simulink model "gm_cosim_fir_mq"  (R2015b)
settings: Solver=FixedStepDiscrete  SolverMode=SingleTasking  StartTime=0.0  StopTime=10.0  RelTol=1e-3
libraries: simulink x2, modelsimlib x1
settings Model: Creator=at-mt  LastModifiedBy=amatsumo
settings DataIOCC: SaveFormat=Array  SignalLoggingSaveFormat=ModelDataLogs  SaveOutput=off  SignalLogging=off  SaveTime=off
settings OptimizationCC: DefaultParameterBehavior=Inlined  ExpressionDepthLimit=2147483647
settings DebuggingCC: AlgebraicLoopMsg=error  UnderspecifiedInitializationDetection=Classic  MergeDetectMultiDrivingBlocksExec=none  SolverPrmCheckMsg=warning  InheritedTsInSrcMsg=none  SingleTaskRateTransMsg=error  ParameterPrecisionLossMsg=none  ParameterTunabilityLossMsg=none  FcnCallInpInsideContextMsg=UseLocalSettings  StateNameClashWarn=warning  StrictBusMsg=Warning
settings HardwareCC: ProdBitPerPointer=32  ProdLargestAtomicFloat=None  ProdIntDivRoundTo=Undefined  ProdEndianess=Unspecified  ProdWordSize=32  ProdHWDeviceType=ASIC/FPGA->ASIC/FPGA  ProdEqTarget=off
settings ModelReferenceCC: UpdateModelReferenceTargets=IfOutOfDate
settings SFSimCC: SFSimEcho=off
settings GRTTargetCC: GeneratePreprocessorConditionals=Disable all  CombineOutputUpdateFcns=off  GRTInterface=on
settings ConfigComp: CovModelRefEnable=Off  CovSFcnEnable=off

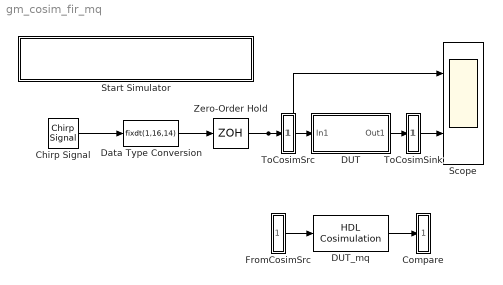
== system gm_cosim_fir_mq ==
  Chirp Signal : simulink/Sources/Chirp Signal  f1=10  T=10  f2=500
  Compare : Subsystem
      mask Display: disp('')
  DUT : Subsystem
  DUT_mq : modelsimlib/HDL Cosimulation  PortPaths=/DUT/In1;/DUT/Out1  PortModes=[1 2 ]  PortTimes="[-1                                                             0.001 ]"  PortSigns=[-1 1 ]  PortFracLengths=[0,14]  CommLocal=on  CommSharedMemory=on  CommPortNumber=4449  CommShowInfo=on  ClockModes=[]  ClockTimes=[]  TclPreSimCommand=|  TclPostSimCommand="puts \"done\""  TimingMode=ns  TimingScaleFactor=10000  idxCellArray={'UNUSED_VAR'}  CosimBypass=Full Simulation  AllowDirectFeedthrough=on  ProductName=EDA Simulator Link MQ  RunAutoTimescale=off  HdlClocks=0  PreRunTime=40  PreRunTimeUnit=ns
      | puts "Running Simulink Cosimulation block.";
      |  puts "Chip Name: --> cosim_fir/DUT";
      |  puts "Target language: --> verilog";
      |  puts "Target directory: --> hdlsrc\cosim_fir";
      |  puts [clock format [clock seconds]];
      | # Clock force command;
      | force /DUT/clk 0 0ns, 1 5ns -r 10ns;
      | # Clock enable force command;
      | force /DUT/clk_enable 0 0ns, 1 37ns;
      | # Reset force command;
      | force /DUT/reset 1 0ns, 0 27ns;
  Data Type Conversion : DataTypeConversion  OutDataTypeStr=fixdt(1,16,14)  RndMeth=Nearest
  FromCosimSrc : Subsystem
      mask Display: disp('')
  Scope : Scope  NumInputPorts=2
  Start Simulator : Subsystem
      settings: OpenFcn=|
      | try
      |    cosimDirName = pwd;
      |    cd 'hdlsrc\cosim_fir';
      |    vsim('tclstart',gm_cosim_fir_mq_tcl);
      |    cd (cosimDirName);
      |    clear cosimDirName;
      | catch me
      |    disp('Failed to launch cosimulator with "vsim"');
      |    disp (me.message);
      |    cd (cosimDirName);
      |    clear cosimDirName;
      | end
      mask Display: disp(['vsimulink work.DUT' char(10) 'Double-click here to launch ModelSim'])
  ToCosimSink : Subsystem
      mask Display: disp('')
  ToCosimSrc : Subsystem
      mask Display: disp('')
  Zero-Order Hold : ZeroOrderHold  SampleTime=1/1000
  wires:
  Chirp Signal/1 -> Data Type Conversion/1
  Zero-Order Hold/1 -> Scope/1, ToCosimSrc/1(in1)
  Data Type Conversion/1 -> Zero-Order Hold/1
  ToCosimSrc/1(out1) -> DUT/1(In1)
  DUT/1(Out1) -> ToCosimSink/1(in1)
  ToCosimSink/1(out1) -> Scope/2
  FromCosimSrc/1(out1) -> DUT_mq/1
  DUT_mq/1 -> Compare/1(in1)

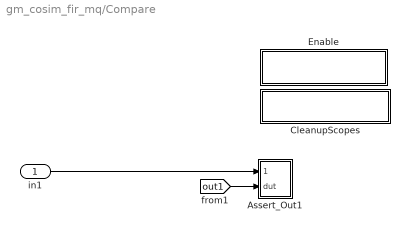
== system gm_cosim_fir_mq/Compare ==
  in1 : Inport
  Assert_Out1 : Subsystem
  CleanupScopes : Subsystem
      settings: OpenFcn=|
      | blkName = gcb;
      | idx = regexp(blkName, '/CleanupScopes$', 'once');
      | blkParent = blkName(1:idx-1);
      | blks=find_system(blkParent, 'blocktype', 'Scope');
      | e = get_param(blks{1}, 'Open');
      | if strcmp(e, 'on'), f= 'off'; else f = 'on'; end
      | for ii=1:length(blks), set_param(blks{ii}, 'Open', f); end; drawnow;
      mask Display: disp(['Double click to\n turn on/off all scopes'])
  Enable : Subsystem
      settings: OpenFcn=|
      | blkName = gcb;
      | idx = regexp(blkName, '/Enable$', 'once');
      | blkParent = blkName(1:idx-1);
      | blks=find_system(blkParent, 'blocktype', 'Assertion');
      | e = get_param(blks{1}, 'Enabled');
      | if strcmp(e, 'on'), f= 'off';, else, f = 'on';, end
      | for ii=1:length(blks), set_param(blks{ii}, 'Enabled', f);, end
      | dispMsg = sprintf('disp([''Double click to turn %s \\n all Assertions''])', upper(e));
      | set_param(gcb, 'MaskDisplay', dispMsg);
      mask Display: disp(['Double click to turn OFF \n all Assertions'])
  wires:
  in1/1 -> Assert_Out1/1(cosim)
  [out1] -> Assert_Out1/2(dut)

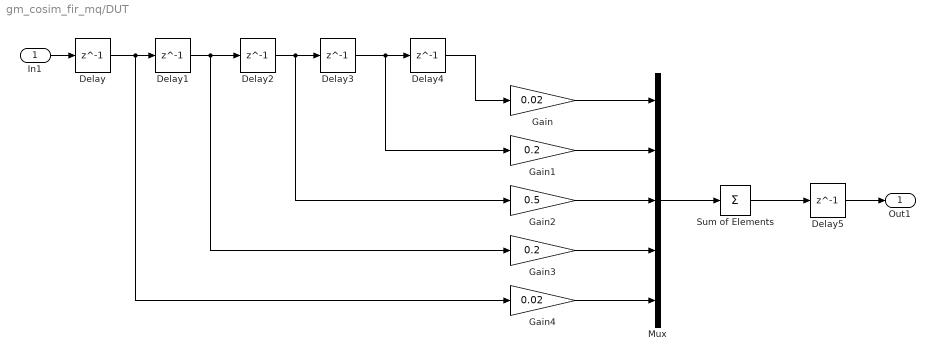
== system gm_cosim_fir_mq/DUT ==
  In1 : Inport
  Delay{,1..5} (6 alike) : Delay  DelayLength=1
  Gain : Gain  Gain=0.02  OutDataTypeStr=Inherit: Same as input
  Gain1 : Gain  Gain=0.2  OutDataTypeStr=Inherit: Same as input
  Gain2 : Gain  Gain=0.5  OutDataTypeStr=Inherit: Same as input
  Gain3 : Gain  Gain=0.2  OutDataTypeStr=Inherit: Same as input
  Gain4 : Gain  Gain=0.02  OutDataTypeStr=Inherit: Same as input
  Mux : Mux  Inputs=5
  Sum of Elements : Sum  Inputs=+
  Out1 : Outport
  wires:
  Sum of Elements/1 -> Delay5/1
  Gain4/1 -> Mux/5
  Gain3/1 -> Mux/4
  Gain2/1 -> Mux/3
  Gain1/1 -> Mux/2
  Gain/1 -> Mux/1
  Mux/1 -> Sum of Elements/1
  In1/1 -> Delay/1
  Delay5/1 -> Out1/1
  Delay1/1 -> Delay2/1, Gain3/1
  Delay2/1 -> Delay3/1, Gain2/1
  Delay3/1 -> Delay4/1, Gain1/1
  Delay4/1 -> Gain/1
  Delay/1 -> Delay1/1, Gain4/1

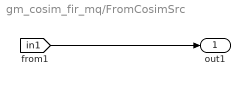
== system gm_cosim_fir_mq/FromCosimSrc ==
  out1 : Outport
  wires:
  [in1] -> out1/1

== system gm_cosim_fir_mq/Start Simulator ==

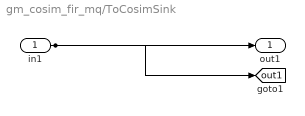
== system gm_cosim_fir_mq/ToCosimSink ==
  in1 : Inport
  out1 : Outport
  tag scope: out1=global
  wires:
  in1/1 -> out1/1, [out1]

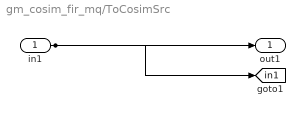
== system gm_cosim_fir_mq/ToCosimSrc ==
  in1 : Inport
  out1 : Outport
  tag scope: in1=global
  wires:
  in1/1 -> out1/1, [in1]

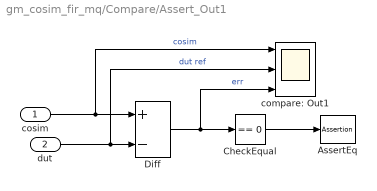
== system gm_cosim_fir_mq/Compare/Assert_Out1 ==
  cosim : Inport
  dut : Inport  Port=2
  AssertEq : Assertion  StopWhenAssertionFail=off
  CheckEqual : simulink/Logic and Bit Operations/Compare To Zero  relop===  OutDataTypeStr=uint8  ZeroCross=off
  Diff : Sum  Inputs=+-
  compare: Out1 : Scope  NumInputPorts=3
  wires:
  CheckEqual/1 -> AssertEq/1
  dut/1 -> Diff/2, compare: Out1/2  "dut ref"
  cosim/1 -> compare: Out1/1, Diff/1  "cosim"
  Diff/1 -> CheckEqual/1, compare: Out1/3  "err"

== system gm_cosim_fir_mq/Compare/CleanupScopes ==

== system gm_cosim_fir_mq/Compare/Enable ==
